simulink model "rollerCoaster"  (R2014a)
settings: Solver=ode45  StartTime=0.0  StopTime=10.0  RelTol=1e-3
settings Model: Creator=tc  LastModifiedBy=tc

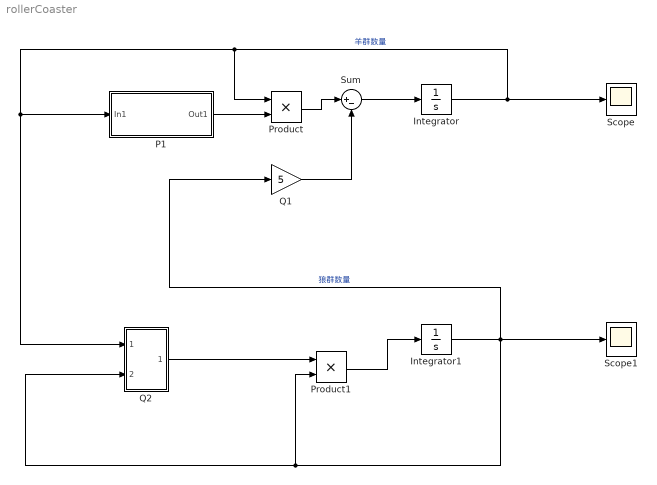
== system rollerCoaster ==
  Integrator : Integrator  InitialCondition=100
  Integrator1 : Integrator  InitialCondition=2
  P1 : Subsystem
  Product : Product
  Product1 : Product
  Q1 : Gain  Gain=5
  Q2 : Subsystem
  Scope : Scope
      settings: TimeRange=10  YMin=0  YMax=200
  Scope1 : Scope
      settings: TimeRange=10  YMin=0  YMax=20
  Sum : Sum  Inputs=|+-
  wires:
  Integrator/1 -> Product/1, Q2/1(In1), P1/1(In1), Scope/1  "羊群数量"
  Integrator1/1 -> Q2/2(In2), Product1/2, Q1/1, Scope1/1  "狼群数量"
  Sum/1 -> Integrator/1
  Product1/1 -> Integrator1/1
  Product/1 -> Sum/1
  P1/1(Out1) -> Product/2
  Q1/1 -> Sum/2
  Q2/1(Out1) -> Product1/1

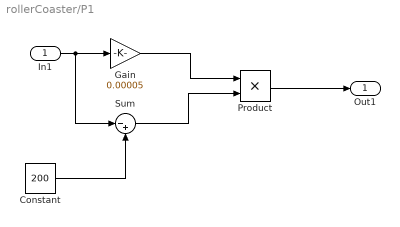
== system rollerCoaster/P1 ==
  In1 : Inport
  Constant : Constant  Value=200
  Gain : Gain  Gain=0.00005
  Product : Product
  Sum : Sum  Inputs=|-+
  Out1 : Outport
  wires:
  In1/1 -> Sum/1, Gain/1
  Constant/1 -> Sum/2
  Gain/1 -> Product/1
  Sum/1 -> Product/2
  Product/1 -> Out1/1

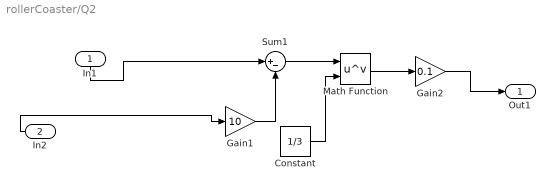
== system rollerCoaster/Q2 ==
  In1 : Inport
  In2 : Inport  Port=2
  Constant : Constant  Value=1/3
  Gain1 : Gain  Gain=10
  Gain2 : Gain  Gain=0.1
  Math Function : Math  Operator=pow  SaturateOnIntegerOverflow=on
  Sum1 : Sum  Inputs=|+-
  Out1 : Outport
  wires:
  Math Function/1 -> Gain2/1
  Constant/1 -> Math Function/2
  In1/1 -> Sum1/1
  Gain1/1 -> Sum1/2
  Sum1/1 -> Math Function/1
  Gain2/1 -> Out1/1
  In2/1 -> Gain1/1
